simulink model "dynamicANN"  (R2019b)
settings: Solver=VariableStepAuto  StartTime=0.0  StopTime=3  RelTol=1e-3
values from neighbouring files (symbols this model uses):
  a = 87.548e-3    (= 0.087548)    [main.m]
  b = 132.452e-3    (= 0.132452)    [main.m]
  d = 22.452e-3    (= 0.022452)    [main.m]
  delta = 4e-6    (= 4e-06)    [main.m]
  F1 = mass*g-F2    (= 23.4474357109)    [main.m]
  F2 = a*mass*g/(a+b)    (= 15.4982642891)    [main.m]
  g = 9.81    [main.m]
  h0 = 75e-6    (= 7.5e-05)    [main.m]
  Jd = 0.047331604    [main.m]
  Jp = 0.00075    [main.m]
  Kps = (Vmax-Vmin)/(Hmax-Hmin)    (= 1666.66666667)    [main.m]
  Ksv = 30    [main.m]
  mass = 3.970    (= 3.97)    [main.m]
  mm = F2/g    (= 1.57984345455)    [main.m]
  omega = n_rpm*2*pi/60    (= 293.215314335)    [main.m]
  s = 30e-3    (= 0.03)    [main.m]
  tau = 0.12    [main.m]
  taus = 0.00125    [main.m]
  Ts = 1/fs    (= 0.001)    [main.m]
libraries: neural x480, simulink x2
(part 6 of 11)

== system dynamicANN/BEARING 2 NL1/B2NN /Layer 2/Delays 1 ==
  "p{2}" : Inport  PortDimensions=100
      mask Display: e = 0.06;c1 = [120 230 180]/255;c2 = ([120 230 180]+0)/(256+128);c3 = ([120 230 180]+128)/(256+128);patch([0 1 1 0],[0 0 1 1],c1);patch([0 1 1 1-e 1-e 0+e],[0 0 1 1-e 0+e 0+e],c2);patch([0 0 1 1-e 0+e 0+e],[0 1 1 1-e 1-e 0+e],c3);plot([0 1 1 0 0],[0 0 1 1 0]);
  mux : Mux  Inputs=1
      mask Display: e = 0.06;c1 = [120 150 230]/255;c2 = ([120 150 230]+0)/383;c3 = ([120 150 230]+128)/383;patch([0 1 1 0],[0 0 1 1],c1);patch([0 1 1 1-e 1-e 0+e],[0 0 1 1-e 0+e 0+e],c2);patch([0 0 1 1-e 0+e 0+e],[0 1 1 1-e 1-e 0+e],c3);plot([0 1 1 0 0],[0 0 1 1 0]);disp('Mux')
  "pd{2,1}" : Outport
      mask Display: e = 0.06;c1 = [120 230 180]/255;c2 = ([120 230 180]+0)/(256+128);c3 = ([120 230 180]+128)/(256+128);patch([0 1 1 0],[0 0 1 1],c1);patch([0 1 1 1-e 1-e 0+e],[0 0 1 1-e 0+e 0+e],c2);patch([0 0 1 1-e 0+e 0+e],[0 1 1 1-e 1-e 0+e],c3);plot([0 1 1 0 0],[0 0 1 1 0]);
  wires:
  "p{2}"/1 -> mux/1
  mux/1 -> "pd{2,1}"/1

== system dynamicANN/BEARING 2 NL1/B2NN /Layer 2/LW{2,1} ==
  "ad{2,1}" : Inport  PortDimensions=100
      mask Display: e = 0.06;c1 = [120 230 180]/255;c2 = ([120 230 180]+0)/(256+128);c3 = ([120 230 180]+128)/(256+128);patch([0 1 1 0],[0 0 1 1],c1);patch([0 1 1 1-e 1-e 0+e],[0 0 1 1-e 0+e 0+e],c2);patch([0 0 1 1-e 0+e 0+e],[0 1 1 1-e 1-e 0+e],c3);plot([0 1 1 0 0],[0 0 1 1 0]);
  "IW{2,1}(1,:)'" : Constant  Value=[1.401049187147146657395069269114173948764801025390625;-0.68586304645464390983278235580655746161937713623046875;0.6748641437408589016655469094985164701938629150390625;1.0066130567927533689953634166158735752105712890625;0.83515429397160778623998567127273418009281158447265625;1.3483440132695012625418939933297224342823028564453125;-0.355073471999288070577449616394005715847015380859375;-2.0688990697969966703340105595998466014862060546875;0.451038999942631468886844459120766259729862213134765625;-1.62961520560310457739205958205275237560272216796875;-1.635704514037160439698936897912062704563140869140625;0.60552191497707286149676519926288165152072906494140625;-1.9439935434929223045941171221784316003322601318359375;-0.2305476851468014343193857484948239289224147796630859375;0.455741450739857445473290908921626396477222442626953125;-0.06422613561783917235370466869426309131085872650146484375;3.1640829742766953813770669512450695037841796875;-1.3892674137189151561955213765031658113002777099609375;1.64364175376021659502612237702123820781707763671875;1.6488052538848754213773872834281064569950103759765625;3.6231436568685726484773113043047487735748291015625;3.3130649985922975275798307848162949085235595703125;0.2180422409655282667273468177882023155689239501953125;-1.0263125270169271008313671700307168066501617431640625;2.473077357550968802257784773246385157108306884765625;-2.377587882090011373037441444466821849346160888671875;0.1291001046565924681441828170136432163417339324951171875;-0.08588615557842592396209369098869501613080501556396484375;-0.660309821590154388815108177368529140949249267578125;-0.377667072912789836269809029545285739004611968994140625;-1.5162820084633015227382202283479273319244384765625;-0.67484624476467691689407502053654752671718597412109375;-0.07741418502305620619186043995796353556215763092041015625;-4.33458489716116535106493756757117807865142822265625;1.69899076235518453614758982439525425434112548828125;-1.0331904761435601880492640702868811786174774169921875;2.01806801412600744782821493572555482387542724609375;1.0953775913315093593070059796446003019809722900390625;-0.5085846251711227949954263749532401561737060546875;0.346826765638977685402011275073164142668247222900390625;3.753364158537937367299264224129728972911834716796875;3.6798644474966710760099886101670563220977783203125;-0.04302906582942622737419924305868335068225860595703125;0.24919921755121798856436043934081681072711944580078125;-0.63074295110169387168497223683516494929790496826171875;-0.5411885911628482315194332841201685369014739990234375;-1.2211024886738537365005186074995435774326324462890625;0.585337278279474571007767735864035785198211669921875;0.2274456796009232395494592537943390198051929473876953125;2.840947710841956297400656694662757217884063720703125;0.3372266991340324704395925436983816325664520263671875;1.0209038593480237455679571212385781109333038330078125;0.47044178412073101025470123204286210238933563232421875;2.854751616918999701510983868502080440521240234375;2.415022768696232891016961730201728641986846923828125;-1.3505430753683393962916170494281686842441558837890625;-1.11633866384169611052357140579260885715484619140625;-1.100183860060094165334021454327739775180816650390625;-2.891741788513237931823596227332018315792083740234375;0.87280176055596891959709182629012502729892730712890625;1.2387844904874409923678513223421759903430938720703125;-1.3699071263094790840142422894132323563098907470703125;3.70892381170641982635061140172183513641357421875;1.4664211496292758329929029059712775051593780517578125;-0.72192825394582926801234634694992564618587493896484375;-0.183565736896078968154455424155457876622676849365234375;-0.7920695727935955776644050274626351892948150634765625;-1.024238964948371855001596486545167863368988037109375;-0.743837530262426493976590791135095059871673583984375;0.43424820286380982903295944197452627122402191162109375;1.067262407493898113131081117899157106876373291015625;1.4791924346817335589321373845450580120086669921875 ...(+1533 chars)]
      mask Display: e = 0.06;c1 = [120 150 230]/255;c2 = ([120 150 230]+0)/383;c3 = ([120 150 230]+128)/383;patch([0 1 1 0],[0 0 1 1],c1);patch([0 1 1 1-e 1-e 0+e],[0 0 1 1-e 0+e 0+e],c2);patch([0 0 1 1-e 0+e 0+e],[0 1 1 1-e 1-e 0+e],c3);plot([0 1 1 0 0],[0 0 1 1 0]);disp('weights');
  "IW{2,1}(2,:)'" : Constant  Value=[-1.34072086313949245806043109041638672351837158203125;3.243160063351574695644785606418736279010772705078125;-0.19519337966432670494754120227298699319362640380859375;0.6854068188202082634319367571151815354824066162109375;0.49865335362349838543849500638316385447978973388671875;-1.73676920449941984969655095483176410198211669921875;1.186826979601851572709847459918819367885589599609375;-0.84640172403323454819457083431188948452472686767578125;-2.97843989699297484463613727712072432041168212890625;2.002384324838466067575382112408988177776336669921875;1.2068293868854207406826617443584837019443511962890625;1.0411221931925371819716019672341644763946533203125;-1.1113979718050586154021175389061681926250457763671875;0.035915300309388574484525946672874852083623409271240234375;-1.7734700873580226954118188587017357349395751953125;2.744111922418405402623875488643534481525421142578125;-1.947555312098206314885828760452568531036376953125;-0.998461123601117161996398863266222178936004638671875;0.720348688552011839902888823417015373706817626953125;2.31629097463152078262282884679734706878662109375;1.7677185295808823806140708256862126290798187255859375;1.621890803638528222307968462700955569744110107421875;1.542041592997760890426661717356182634830474853515625;-0.9572617828775962234288954277872107923030853271484375;-1.991011962767576193300556042231619358062744140625;-2.1518752218119789887396109406836330890655517578125;-0.87432723839731563142407821942470036447048187255859375;3.288679052536858105071360114379785954952239990234375;-0.9944905705817472796326228490215726196765899658203125;1.1209860854108910643844865262508392333984375;4.0697217365483169260187423788011074066162109375;2.6416877338926649798622747766785323619842529296875;0.1682343583399872610772973757775616832077503204345703125;3.035862993161661638197301726904697716236114501953125;1.9209902390411286443594462980399839580059051513671875;-0.90509709317922404370193589784321375191211700439453125;-0.405486953924359294632040473516099154949188232421875;-0.640243742992463893415333586744964122772216796875;1.829343984262926436912266581202857196331024169921875;1.6237283050980539922392154039698652923107147216796875;-3.59170411269922684738276075222529470920562744140625;3.541688637154810859186682137078605592250823974609375;0.465557163002664198270252882139175198972225189208984375;0.1883293542782208118691045228842995129525661468505859375;-0.659082172058047977003525375039316713809967041015625;2.004836797370756595881857720087282359600067138671875;-0.46208591707920987357027797770570032298564910888671875;3.2519247773882380414534054580144584178924560546875;0.6096465282952951980632860795594751834869384765625;1.6821838045840629138893973504309542477130889892578125;-2.601200708982287057580151667934842407703399658203125;1.50413812343383579417377404752187430858612060546875;-0.0354886306454344213623386394829140044748783111572265625;-2.5602762535924181719337866525165736675262451171875;-1.5312265030995815262571113635203801095485687255859375;-2.27670917114064508268711506389081478118896484375;2.912571648930722734149867392261512577533721923828125;3.23264693866010599521132462541572749614715576171875;-2.52674619181376858279008956742472946643829345703125;0.2136113293922726474871609525507665239274501800537109375;2.752698221459216387785318147507496178150177001953125;-1.4269405021043013448434066958725452423095703125;1.8467803076175623999688468757085502147674560546875;0.53629363236735760889217772273696027696132659912109375;-0.9025095252280930235855294085922650992870330810546875;2.3965941110137141123459514346905052661895751953125;-0.440612566468998101409937362404889427125453948974609375;1.5845732918717361226157436249195598065853118896484375;5.518651706014896518581736017949879169464111328125;0.7622345517031117179129751093569211661815643310546875;-1.887983696220212781469172114157117903232574462890625;0.80728662951480167908613339022849686443805694580078125;-0.0703367258630312186529209839136456139385700225830078125 ...(+1486 chars)]
      mask Display: e = 0.06;c1 = [120 150 230]/255;c2 = ([120 150 230]+0)/383;c3 = ([120 150 230]+128)/383;patch([0 1 1 0],[0 0 1 1],c1);patch([0 1 1 1-e 1-e 0+e],[0 0 1 1-e 0+e 0+e],c2);patch([0 0 1 1-e 0+e 0+e],[0 1 1 1-e 1-e 0+e],c3);plot([0 1 1 0 0],[0 0 1 1 0]);disp('weights');
  Mux : Mux  Inputs=2
      mask Display: e = 0.06;c1 = [120 150 230]/255;c2 = ([120 150 230]+0)/383;c3 = ([120 150 230]+128)/383;patch([0 1 1 0],[0 0 1 1],c1);patch([0 1 1 1-e 1-e 0+e],[0 0 1 1-e 0+e 0+e],c2);patch([0 0 1 1-e 0+e 0+e],[0 1 1 1-e 1-e 0+e],c3);plot([0 1 1 0 0],[0 0 1 1 0]);disp('Mux');
  dotprod1 : neural/Weight Functions/dotprod
      settings: SourceProductName=Deep Learning Toolbox
  dotprod2 : neural/Weight Functions/dotprod
      settings: SourceProductName=Deep Learning Toolbox
  "lz{2,1}" : Outport
      mask Display: e = 0.06;c1 = [120 230 180]/255;c2 = ([120 230 180]+0)/(256+128);c3 = ([120 230 180]+128)/(256+128);patch([0 1 1 0],[0 0 1 1],c1);patch([0 1 1 1-e 1-e 0+e],[0 0 1 1-e 0+e 0+e],c2);patch([0 0 1 1-e 0+e 0+e],[0 1 1 1-e 1-e 0+e],c3);plot([0 1 1 0 0],[0 0 1 1 0]);
  wires:
  "IW{2,1}(1,:)'"/1 -> dotprod1/1
  "ad{2,1}"/1 -> dotprod1/2, dotprod2/2
  dotprod1/1 -> Mux/1
  "IW{2,1}(2,:)'"/1 -> dotprod2/1
  dotprod2/1 -> Mux/2
  Mux/1 -> "lz{2,1}"/1

== system dynamicANN/ROTOR SYSTEM WITH ANN1/B1NN/Layer 1/Delays 1 ==
  "p{1}" : Inport  PortDimensions=4
      mask Display: e = 0.06;c1 = [120 230 180]/255;c2 = ([120 230 180]+0)/(256+128);c3 = ([120 230 180]+128)/(256+128);patch([0 1 1 0],[0 0 1 1],c1);patch([0 1 1 1-e 1-e 0+e],[0 0 1 1-e 0+e 0+e],c2);patch([0 0 1 1-e 0+e 0+e],[0 1 1 1-e 1-e 0+e],c3);plot([0 1 1 0 0],[0 0 1 1 0]);
  mux : Mux  Inputs=1
      mask Display: e = 0.06;c1 = [120 150 230]/255;c2 = ([120 150 230]+0)/383;c3 = ([120 150 230]+128)/383;patch([0 1 1 0],[0 0 1 1],c1);patch([0 1 1 1-e 1-e 0+e],[0 0 1 1-e 0+e 0+e],c2);patch([0 0 1 1-e 0+e 0+e],[0 1 1 1-e 1-e 0+e],c3);plot([0 1 1 0 0],[0 0 1 1 0]);disp('Mux')
  "pd{1,1}" : Outport
      mask Display: e = 0.06;c1 = [120 230 180]/255;c2 = ([120 230 180]+0)/(256+128);c3 = ([120 230 180]+128)/(256+128);patch([0 1 1 0],[0 0 1 1],c1);patch([0 1 1 1-e 1-e 0+e],[0 0 1 1-e 0+e 0+e],c2);patch([0 0 1 1-e 0+e 0+e],[0 1 1 1-e 1-e 0+e],c3);plot([0 1 1 0 0],[0 0 1 1 0]);
  wires:
  "p{1}"/1 -> mux/1
  mux/1 -> "pd{1,1}"/1
